simulink library "PB_Library_Master_Working"  (R2021a)
settings: Solver=VariableStepAuto  StartTime=0.0  StopTime=10.0  RelTol=1e-3
undefined symbols (not defined in the file): A_M, B_M, component_degradation_input, E0_M, f_sw, f_sw_M_aDF, flux_m_aDF, Fsw_M_aDF, insert, K_M, L_M_aDF, L_M_adf, P_Fe_Nom_aDF, Q_M, Q_rr, r_c, r_D, R_M, R_s_aDF, resistance_aDF, S_nom_aDF, SOC_Init_M, TFall_M_aDF, TRise_M_aDF, Trr_M_aDF, u_ce0, u_D0
libraries: $bdroot x76, Lib_Dyn_StateSpace_EMTAT x6, Lib_PF_BusLoadDC_TMATS x3, PB_Library_Master x3, simulink x3, TemperatureBlock x1
(part 5 of 5)

== system PB_Library_Master_Working/Boost Converter/DC - DC Converter/Steady State/TemperatureModifiedPerformanceTerm1 /TModifiedROn  ==
  In1 : Inport
  Add4 : Sum
  Constant10 : Constant  Value=50
  Constant9 : Constant  Value=25
  Divide : Product  Inputs=*/
  Multiply : Product
  "OnResistance " : Constant  Value=Ron_M
  Out1 : Outport  VectorParamsAs1DForOutWhenUnconnected=off
  wires:
  In1/1 -> Add4/1
  Constant10/1 -> Divide/2
  Add4/1 -> Divide/1
  Constant9/1 -> Add4/2
  Divide/1 -> Multiply/2
  Multiply/1 -> Out1/1
  "OnResistance "/1 -> Multiply/1

== system PB_Library_Master_Working/Boost Converter/DC - DC Converter/Steady State/TemperatureModifiedPerformanceTerm2 /TModifiedROn  ==
  In1 : Inport
  Add4 : Sum
  Constant10 : Constant  Value=50
  Constant9 : Constant  Value=25
  Divide : Product  Inputs=*/
  Multiply : Product
  "OnResistance " : Constant  Value=Ron_M
  Out1 : Outport  VectorParamsAs1DForOutWhenUnconnected=off
  wires:
  In1/1 -> Add4/1
  Constant10/1 -> Divide/2
  Add4/1 -> Divide/1
  Constant9/1 -> Add4/2
  Divide/1 -> Multiply/2
  Multiply/1 -> Out1/1
  "OnResistance "/1 -> Multiply/1

== system PB_Library_Master_Working/Boost Converter Analytic/DC - DC Converter/Steady State/TemperatureModifiedPerformanceTerm1 /TModifiedROn  ==
  In1 : Inport
  Add4 : Sum
  Constant10 : Constant  Value=50
  Constant9 : Constant  Value=25
  Divide : Product  Inputs=*/
  Multiply : Product
  "OnResistance " : Constant  Value=Ron_M
  Out1 : Outport  VectorParamsAs1DForOutWhenUnconnected=off
  wires:
  In1/1 -> Add4/1
  Constant10/1 -> Divide/2
  Add4/1 -> Divide/1
  Constant9/1 -> Add4/2
  Divide/1 -> Multiply/2
  Multiply/1 -> Out1/1
  "OnResistance "/1 -> Multiply/1

== system PB_Library_Master_Working/Boost Converter Analytic/DC - DC Converter/Steady State/TemperatureModifiedPerformanceTerm2 /TModifiedROn  ==
  In1 : Inport
  Add4 : Sum
  Constant10 : Constant  Value=50
  Constant9 : Constant  Value=25
  Divide : Product  Inputs=*/
  Multiply : Product
  "OnResistance " : Constant  Value=Ron_M
  Out1 : Outport  VectorParamsAs1DForOutWhenUnconnected=off
  wires:
  In1/1 -> Add4/1
  Constant10/1 -> Divide/2
  Add4/1 -> Divide/1
  Constant9/1 -> Add4/2
  Divide/1 -> Multiply/2
  Multiply/1 -> Out1/1
  "OnResistance "/1 -> Multiply/1

== system PB_Library_Master_Working/Buck Converter/DC - DC Converter/Steady State/TemperatureModifiedPerformanceTerm2 /TModifiedROn  ==
  In1 : Inport
  Add4 : Sum
  Constant10 : Constant  Value=50
  Constant9 : Constant  Value=25
  Divide : Product  Inputs=*/
  Multiply : Product
  "OnResistance " : Constant  Value=Ron_M
  Out1 : Outport  VectorParamsAs1DForOutWhenUnconnected=off
  wires:
  In1/1 -> Add4/1
  Constant10/1 -> Divide/2
  Add4/1 -> Divide/1
  Constant9/1 -> Add4/2
  Divide/1 -> Multiply/2
  Multiply/1 -> Out1/1
  "OnResistance "/1 -> Multiply/1

== system PB_Library_Master_Working/Buck Converter Analytic/DC - DC Converter/Steady State/TemperatureModifiedPerformanceTerm2 /TModifiedROn  ==
  In1 : Inport
  Add4 : Sum
  Constant10 : Constant  Value=50
  Constant9 : Constant  Value=25
  Divide : Product  Inputs=*/
  Multiply : Product
  "OnResistance " : Constant  Value=Ron_M
  Out1 : Outport  VectorParamsAs1DForOutWhenUnconnected=off
  wires:
  "OnResistance "/1 -> Multiply/1
  Multiply/1 -> Out1/1
  Divide/1 -> Multiply/2
  Constant9/1 -> Add4/2
  Add4/1 -> Divide/1
  Constant10/1 -> Divide/2
  In1/1 -> Add4/1

== matlab function PB_Library_Master_Working/Boost Converter/DC - DC Converter/MATLAB Function ==
  data: A1 input; y output; dt input
function y  = switchLogic(A1, dt)    %A1 state martix, dt time step    

StableFlag=all(abs(1+dt*eig(A1))<=1);    %Forward Euler Stability requirement

if StableFlag==1
    y=1;    %runs dynamic model
    
else
    y=0;    %runs steady state model
    
end

end

== matlab function PB_Library_Master_Working/Buck Converter/DC - DC Converter/MATLAB Function ==
  data: A1 input; y output; dt input
function y  = switchLogic(A1, dt)    %A1 state martix, dt time step    

StableFlag=all(abs(1+dt*eig(A1))<=1);    %Forward Euler Stability requirement

if StableFlag==1
    y=1;    %runs dynamic model
    
else
    y=0;    %runs steady state model
    
end

end

== matlab function PB_Library_Master_Working/Buck Converter Analytic/DC - DC Converter/MATLAB Function ==
  data: A1 input; y output; dt input
function y  = switchLogic(A1, dt)    %A1 state martix, dt time step    

StableFlag=all(abs(1+dt*eig(A1))<=1);    %Forward Euler Stability requirement

if StableFlag==1
    y=1;    %runs dynamic model
    
else
    y=0;    %runs steady state model
    
end

end

== matlab function PB_Library_Master_Working/Boost Converter Analytic/DC - DC Converter/MATLAB Function ==
  data: A1 input; y output; dt input
function y  = switchLogic(A1, dt)    %A1 state martix, dt time step    

StableFlag=all(abs(1+dt*eig(A1))<=1);    %Forward Euler Stability requirement

if StableFlag==1
    y=1;    %runs dynamic model
    
else
    y=0;    %runs steady state model
    
end

end
